simulink model "OMAP_ver_MIL10"  (R2018b)
settings: Solver=FixedStepDiscrete  StartTime=0.0  StopTime=10.0  FixedStep=0.01  RelTol=1e-3
undefined symbols (not defined in the file or in its folder): OMAP_Switch_EMS, OMAP_Switch_EPS, OMAP_Switch_ESC, OMAP_Switch_IC, OMAP_Switch_OTHER, TH_HMIClb_tiDgrdIconWarnHiDurT_C, TH_HMIClb_tiDgrdIconWarnLoDurT_C, TH_HMIClb_tiDgrdVocWarnDurT_C, TH_HMIClb_tiHndOffTxtWarnT_C, TH_HMIClb_tiHndOffVocWarnT_C, TH_HMIClb_tiSWALimFlgDetT_C, TH_HMIClb_tiTxtLimT_C
libraries: simulink x118
(part 5 of 9)

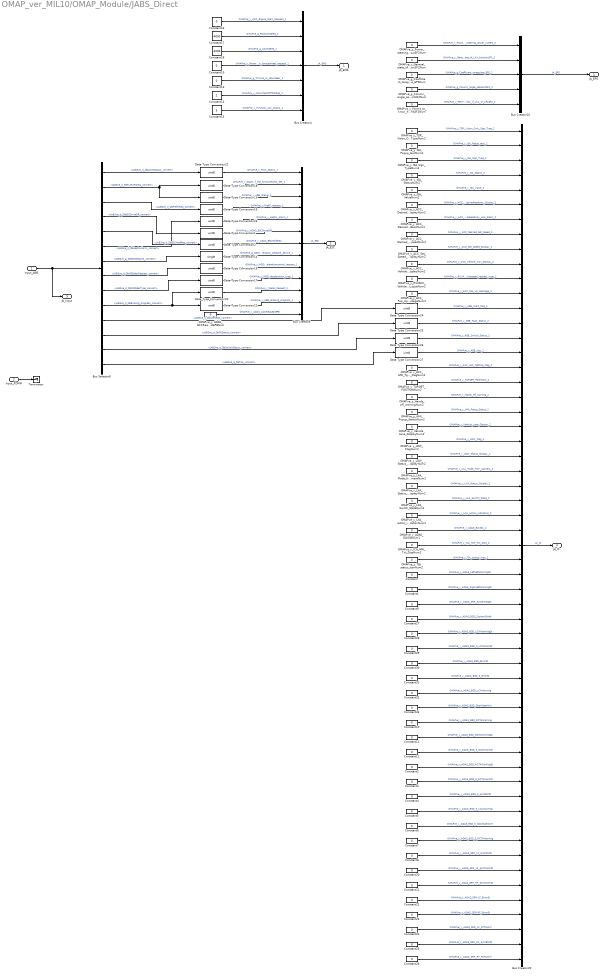
== system OMAP_ver_MIL10/OMAP_Module/JABS_Direct ==
  Input_JABS : Inport
  Input_FDMM : Inport  Port=2
  Bus Creator10 : BusCreator  Inputs=5
  Bus Creator20 : BusCreator  Inputs=57
  Bus Creator4 : BusCreator  Inputs=7
  Bus Creator9 : BusCreator  Inputs=13
  Bus Selector8 : BusSelector  OutputSignals=JABSve_d_DbJACWStatus_convert,JABSve_d_DbFunFARCSta_convert,JABSve_d_DbPrefillReq_convert,JABSve_d_DbESCDriveOff_convert,JABSve_d_DbESCHoldReq_convert,JABSve_d_DbHapticAlarm_convert,JABSve_g_DbDecSetpoint_convert,JABSve_d_DbMDDdecRequest_convert,JABSve_d_DbMDDdecType_convert,JABSve_d_DbBraking_progress_convert,JABSve_d_DbAlertReq_convert,JABSve_d_DbFltStatus_convert,JABSve_d_DbSwitchStatus_convert,JABSve_d_DbTips_convert
  Constant{,1..12,16,19..33} (29 alike) : Constant  Value=0  OutDataTypeStr=uint8
  Constant13 : Constant  Value=0  OutDataTypeStr=single
  Constant14 : Constant  Value=2  OutDataTypeStr=uint8
  Constant15 : Constant  Value=3  OutDataTypeStr=uint8
  Constant17 : Constant  Value=-4000  OutDataTypeStr=single
  Constant18 : Constant  Value=-4000  OutDataTypeStr=single
  Data Type Conversion{1..2,15..27} (15 alike) : DataTypeConversion  OutDataTypeStr=uint8
  Data Type Conversion14 : DataTypeConversion  OutDataTypeStr=single
  OMAPve_g_Coefficient_toregulate_EPSNum : Constant  Value=0  OutDataTypeStr=single
  OMAPve_g_Column_angle_setpoint3F2Num : Constant  Value=0  OutDataTypeStr=single
  OMAPve_y_ACC_DesiredHeadway_DisplayNum2 : Constant  Value=0  OutDataTypeStr=uint8
  OMAPve_y_ACC_DesiredHeadway_Icon_BasicNum2 : Constant  Value=0  OutDataTypeStr=uint8
  OMAPve_y_ACC_Desired_Set_SpeedNum2 : Constant  Value=0  OutDataTypeStr=uint8
  OMAPve_y_ACC_HMI_TgtDisp_FlagNum2 : Constant  Value=0  OutDataTypeStr=uint8
  OMAPve_y_ACC_Pop_Up_MessageNum2 : Constant  Value=0  OutDataTypeStr=uint8
  OMAPve_y_ACC_Set_Speed_DisplayNum2 : Constant  Value=0  OutDataTypeStr=uint8
  OMAPve_y_ACC_Vehicle_Icon_DisplayNum2 : Constant  Value=0  OutDataTypeStr=uint8
  OMAPve_y_ADAS_ACCRequestEPBNum : Constant  Value=0  OutDataTypeStr=uint8
  OMAPve_y_ADAS_ELKStsNum1 : Constant  Value=0  OutDataTypeStr=uint8
  OMAPve_y_General_state_of_LKA_function3F2Num : Constant  Value=0  OutDataTypeStr=uint8
  OMAPve_y_HMI_Popup_StatusNum2 : Constant  Value=0  OutDataTypeStr=uint8
  OMAPve_y_Hands_off_warningNum2 : Constant  Value=0  OutDataTypeStr=uint8
  OMAPve_y_ICA_HMI_Txt_DispNum2 : Constant  Value=0  OutDataTypeStr=uint8
  OMAPve_y_ISA_Popup_textNum2 : Constant  Value=0  OutDataTypeStr=uint8
  OMAPve_y_ISA_Sign_TypeNum2 : Constant  Value=0  OutDataTypeStr=uint8
  OMAPve_y_ISA_StatusNum2 : Constant  Value=0  OutDataTypeStr=uint8
  OMAPve_y_ISA_ValueNum2 : Constant  Value=0  OutDataTypeStr=uint8
  OMAPve_y_LDW_FlagNum2 : Constant  Value=0  OutDataTypeStr=uint8
  OMAPve_y_LDW_Status_DisplayNum2 : Constant  Value=0  OutDataTypeStr=uint8
  OMAPve_y_LKA_Mode_from_CameraNum2 : Constant  Value=0  OutDataTypeStr=uint8
  OMAPve_y_LKA_Status_DisplayNum2 : Constant  Value=0  OutDataTypeStr=uint8
  OMAPve_y_LKA_Switch_StateNum2 : Constant  Value=0  OutDataTypeStr=uint8
  OMAPve_y_LKA_action_indicationNum2 : Constant  Value=0  OutDataTypeStr=uint8
  OMAPve_y_Permit_to_know_if_LKA_or_LPA3F2Num : Constant  Value=0  OutDataTypeStr=uint8
  OMAPve_y_Power_steering_power_cut3F2Num : Constant  Value=0  OutDataTypeStr=uint8
  OMAPve_y_RVVACC_Vehiclespeed_request_typeNum2 : Constant  Value=0  OutDataTypeStr=uint8
  OMAPve_y_TARGET_POSITIONNum2 : Constant  Value=6  OutDataTypeStr=uint8
  OMAPve_y_TJA_status_iconNum2 : Constant  Value=0  OutDataTypeStr=uint8
  OMAPve_y_TSR_Vision_Only_Sign_TypeNum2 : Constant  Value=0  OutDataTypeStr=uint8
  OMAPve_y_Vehicle_Lane_DisplayNum2 : Constant  Value=0  OutDataTypeStr=uint8
  Terminator : Terminator
  JA_EMS : Outport
  JA_ESC : Outport  Port=2
  JA_EPS : Outport  Port=3
  JA_IC : Outport  Port=4
  JA_Input : Outport  Port=5
  wires:
  Bus Creator20/1 -> JA_IC/1  "JA_IC"
  OMAPve_y_ISA_StatusNum2/1 -> Bus Creator20/4  "OMAPve_y_ISA_Status_2"
  Bus Selector8/13 -> Data Type Conversion26/1  "<JABSve_d_DbSwitchStatus_convert>"
  Bus Selector8/14 -> Data Type Conversion27/1  "<JABSve_d_DbTips_convert>"
  Bus Selector8/9 -> Data Type Conversion17/1  "<JABSve_d_DbMDDdecType_convert>"
  Data Type Conversion27/1 -> Bus Creator20/16  "OMAPve_y_AEB_tips_2"
  OMAPve_y_ICA_HMI_Txt_DispNum2/1 -> Bus Creator20/29  "OMAPve_y_ICA_HMI_Txt_Disp_2"
  OMAPve_y_TARGET_POSITIONNum2/1 -> Bus Creator20/18  "OMAPve_y_TARGET_POSITION_2"
  OMAPve_y_ACC_Vehicle_Icon_DisplayNum2/1 -> Bus Creator20/10  "OMAPve_y_ACC_Vehicle_Icon_Display_2"
  Bus Selector8/6 -> Data Type Conversion23/1  "<JABSve_d_DbHapticAlarm_convert>"
  OMAPve_y_HMI_Popup_StatusNum2/1 -> Bus Creator20/20  "OMAPve_y_HMI_Popup_Status_2"
  OMAPve_y_LKA_Status_DisplayNum2/1 -> Bus Creator20/25  "OMAPve_y_LKA_Status_Display_2"
  OMAPve_y_ACC_DesiredHeadway_DisplayNum2/1 -> Bus Creator20/6  "OMAPve_y_ACC_DesiredHeadway_Display_2"
  Data Type Conversion25/1 -> Bus Creator20/14  "OMAPve_y_AEB_Fault_Status_2"
  Data Type Conversion24/1 -> Bus Creator20/13  "OMAPve_y_AEB_Alert_Req_2"
  OMAPve_y_ACC_HMI_TgtDisp_FlagNum2/1 -> Bus Creator20/17  "OMAPve_y_ACC_HMI_TgtDisp_Flag_2"
  Input_JABS/1 -> JA_Input/1, Bus Selector8/1
  OMAPve_y_ISA_Popup_textNum2/1 -> Bus Creator20/2  "OMAPve_y_ISA_Popup_text_2"
  OMAPve_y_LKA_Mode_from_CameraNum2/1 -> Bus Creator20/24  "OMAPve_y_LKA_Mode_from_Camera_2"
  OMAPve_y_ISA_Sign_TypeNum2/1 -> Bus Creator20/3  "OMAPve_y_ISA_Sign_Type_2"
  Bus Selector8/11 -> Data Type Conversion24/1  "<JABSve_d_DbAlertReq_convert>"
  OMAPve_y_Vehicle_Lane_DisplayNum2/1 -> Bus Creator20/21  "OMAPve_y_Vehicle_Lane_Display_2"
  OMAPve_y_LKA_action_indicationNum2/1 -> Bus Creator20/27  "OMAPve_y_LKA_action_indication_2"
  Bus Selector8/1 -> Data Type Conversion22/1  "<JABSve_d_DbJACWStatus_convert>"
  Data Type Conversion15/1 -> Bus Creator9/9  "OMAPve_y_MDD_Decelerationcontrol_request_1"
  OMAPve_y_ACC_Desired_Set_SpeedNum2/1 -> Bus Creator20/8  "OMAPve_y_ACC_Desired_Set_Speed_2"
  OMAPve_y_TSR_Vision_Only_Sign_TypeNum2/1 -> Bus Creator20/1  "OMAPve_y_TSR_Vision_Only_Sign_Type_2"
  Constant15/1 -> Bus Creator4/7  "OMAPve_y_Function_Acc_status_1"
  Bus Creator4/1 -> JA_EMS/1  "JA_EMS"
  Constant13/1 -> Bus Creator4/5  "OMAPve_g_TminUp_or_downGear_1"
  Bus Selector8/12 -> Data Type Conversion25/1  "<JABSve_d_DbFltStatus_convert>"
  OMAPve_y_LDW_Status_DisplayNum2/1 -> Bus Creator20/23  "OMAPve_y_LDW_Status_Display_2"
  Data Type Conversion26/1 -> Bus Creator20/15  "OMAPve_y_AEB_Switch_Status_2"
  Data Type Conversion22/1 -> Bus Creator9/1  "OMAPve_y_FCW_Status_1"
  Data Type Conversion17/1 -> Bus Creator9/10  "OMAPve_y_MDD_deceleration_type_1"
  Data Type Conversion14/1 -> Bus Creator9/8  "OMAPve_g_Deceleration_setpoint_device_1"
  Bus Selector8/3 -> Data Type Conversion16/1  "<JABSve_d_DbPrefillReq_convert>"
  Constant14/1 -> Bus Creator4/6  "OMAPve_y_stAcvTqWhlPTPotReq_1"
  Bus Selector8/8 -> Data Type Conversion15/1  "<JABSve_d_DbMDDdecRequest_convert>"
  Bus Creator9/1 -> JA_ESC/1  "JA_ESC"
  Constant16/1 -> Bus Creator4/1  "OMAPve_y_ACC_Engine_Start_Request_1"
  OMAPve_y_LKA_Switch_StateNum2/1 -> Bus Creator20/26  "OMAPve_y_LKA_Switch_State_2"
  OMAPve_y_ACC_DesiredHeadway_Icon_BasicNum2/1 -> Bus Creator20/7  "OMAPve_y_ACC_DesiredHeadway_Icon_Basic_2"
  OMAPve_y_LDW_FlagNum2/1 -> Bus Creator20/22  "OMAPve_y_LDW_Flag_2"
  Data Type Conversion16/1 -> Bus Creator9/4  "OMAPve_y_Prefill_request_1"
  Data Type Conversion18/1 -> Bus Creator9/2  "OMAPve_y_State_of_the_functionFARC_det_1"
  Constant19/1 -> Bus Creator4/4  "OMAPve_y_Powertrain_torquewheel_request_1"
  OMAPve_y_ISA_ValueNum2/1 -> Bus Creator20/5  "OMAPve_y_ISA_Value_2"
  Data Type Conversion23/1 -> Bus Creator9/5  "OMAPve_y_Haptic_Alarm_1"
  Data Type Conversion19/1 -> Bus Creator9/3  "OMAPve_y_AEB_Status_1"
  OMAPve_y_RVVACC_Vehiclespeed_request_typeNum2/1 -> Bus Creator20/11  "OMAPve_y_RVVACC_Vehiclespeed_request_type_2"
  Bus Selector8/7 -> Data Type Conversion14/1  "<JABSve_g_DbDecSetpoint_convert>"
  Constant18/1 -> Bus Creator4/3  "OMAPve_g_ACCTqReq_1"
  OMAPve_y_Hands_off_warningNum2/1 -> Bus Creator20/19  "OMAPve_y_Hands_off_warning_2"
  OMAPve_y_TJA_status_iconNum2/1 -> Bus Creator20/30  "OMAPve_y_TJA_status_icon_2"
  Constant17/1 -> Bus Creator4/2  "OMAPve_g_PotACCTqReq_1"
  OMAPve_y_ACC_Pop_Up_MessageNum2/1 -> Bus Creator20/12  "OMAPve_y_ACC_Pop_Up_Message_2"
  Bus Selector8/2 -> Data Type Conversion18/1, Data Type Conversion19/1  "<JABSve_d_DbFunFARCSta_convert>"
  Data Type Conversion20/1 -> Bus Creator9/11  "OMAPve_y_Decel_Request_1"
  OMAPve_y_ACC_Set_Speed_DisplayNum2/1 -> Bus Creator20/9  "OMAPve_y_ACC_Set_Speed_Display_2"
  Data Type Conversion21/1 -> Bus Creator9/12  "OMAPve_y_AEB_Braking_progress_1"
  OMAPve_y_Power_steering_power_cut3F2Num/1 -> Bus Creator10/1  "OMAPve_y_Power_steering_power_cut3F2_2"
  Bus Creator10/1 -> JA_EPS/1  "JA_EPS"
  OMAPve_y_Permit_to_know_if_LKA_or_LPA3F2Num/1 -> Bus Creator10/5  "OMAPve_y_Permit_to_know_if_LKA_or_LPA3F2_2"
  OMAPve_g_Coefficient_toregulate_EPSNum/1 -> Bus Creator10/3  "OMAPve_g_Coefficient_toregulate_EPS_2"
  OMAPve_y_General_state_of_LKA_function3F2Num/1 -> Bus Creator10/2  "OMAPve_y_General_state_of_LKA_function3F2_2"
  OMAPve_g_Column_angle_setpoint3F2Num/1 -> Bus Creator10/4  "OMAPve_g_Column_angle_setpoint3F2_2"
  Bus Selector8/10 -> Data Type Conversion20/1, Data Type Conversion21/1  "<JABSve_d_DbBraking_progress_convert>"
  Input_FDMM/1 -> Terminator/1
  OMAPve_y_ADAS_ELKStsNum1/1 -> Bus Creator20/28  "OMAPve_y_ADAS_ELKSts_2"
  Data Type Conversion2/1 -> Bus Creator9/7  "OMAPve_y_ADAS_ESCHoldReq"
  Data Type Conversion1/1 -> Bus Creator9/6  "OMAPve_y_ADAS_ESCDriveOff"
  OMAPve_y_ADAS_ACCRequestEPBNum/1 -> Bus Creator9/13  "OMAPve_y_ADAS_ACCRequestEPB"
  Constant6/1 -> Bus Creator20/48  "OMAPve_y_ADAS_BSD_S_DoorOpenWrn"
  Constant5/1 -> Bus Creator20/47  "OMAPve_y_ADAS_BSD_S_LCAWarning"
  Constant1/1 -> Bus Creator20/32  "OMAPve_y_ADAS_RighrLEDWarningSt"
  Constant8/1 -> Bus Creator20/50  "OMAPve_y_ADAS_SRR_LF_SystStInfo"
  Constant10/1 -> Bus Creator20/41  "OMAPve_y_ADAS_BSD_RCTAWarning"
  Constant33/1 -> Bus Creator20/40  "OMAPve_y_ADAS_BSD_DoorOpenWrn"
  Constant22/1 -> Bus Creator20/53  "OMAPve_y_ADAS_SRR-LF_ErrorSt"
  Constant7/1 -> Bus Creator20/49  "OMAPve_y_ADAS_BSD_S_RCTAWarning"
  Constant20/1 -> Bus Creator20/51  "OMAPve_y_ADAS_SRR_LF_SystWorkSt"
  Constant21/1 -> Bus Creator20/52  "OMAPve_y_ADAS_SRR_RF_SystWorkSt"
  Constant4/1 -> Bus Creator20/46  "OMAPve_y_ADAS_BSD_S_SystStInfo"
  Constant3/1 -> Bus Creator20/45  "OMAPve_y_ADAS_BSD_S_RCTAWorkSt"
  Constant2/1 -> Bus Creator20/44  "OMAPve_y_ADAS_BSD_RCTAWorkingSt"
  Constant23/1 -> Bus Creator20/54  "OMAPve_y_ADAS_SRR-RF_ErrorSt"
  Constant26/1 -> Bus Creator20/57  "OMAPve_y_ADAS_SRR_RF_FCTAWrn"
  Constant/1 -> Bus Creator20/31  "OMAPve_y_ADAS_LeftLEDWarningSt"
  Constant25/1 -> Bus Creator20/56  "OMAPve_y_ADAS_SRR_RF_SystStInfo"
  Constant24/1 -> Bus Creator20/55  "OMAPve_y_ADAS_SRR_LF_FCTAWrn"
  Constant28/1 -> Bus Creator20/35  "OMAPve_y_ADAS_BSD_LCWWorkingSt"
  Constant32/1 -> Bus Creator20/39  "OMAPve_y_ADAS_BSD_LCAWarning"
  Constant12/1 -> Bus Creator20/43  "OMAPve_y_ADAS_BSD_S_DOWWorkSt"
  Constant29/1 -> Bus Creator20/36  "OMAPve_y_ADAS_BSD_S_LCWWorkSt"
  Constant31/1 -> Bus Creator20/38  "OMAPve_y_ADAS_BSD_S_ErrorSt"
  Constant9/1 -> Bus Creator20/33  "OMAPve_y_ADAS_SRR_SystemState"
  Constant30/1 -> Bus Creator20/37  "OMAPve_y_ADAS_BSD_ErrorSt"
  Constant27/1 -> Bus Creator20/34  "OMAPve_y_ADAS_BSD_SystemStInfo"
  Constant11/1 -> Bus Creator20/42  "OMAPve_y_ADAS_BSD_DOWWorkingSt"
  Bus Selector8/4 -> Data Type Conversion1/1  "<JABSve_d_DbESCDriveOff_convert>"
  Bus Selector8/5 -> Data Type Conversion2/1  "<JABSve_d_DbESCHoldReq_convert>"

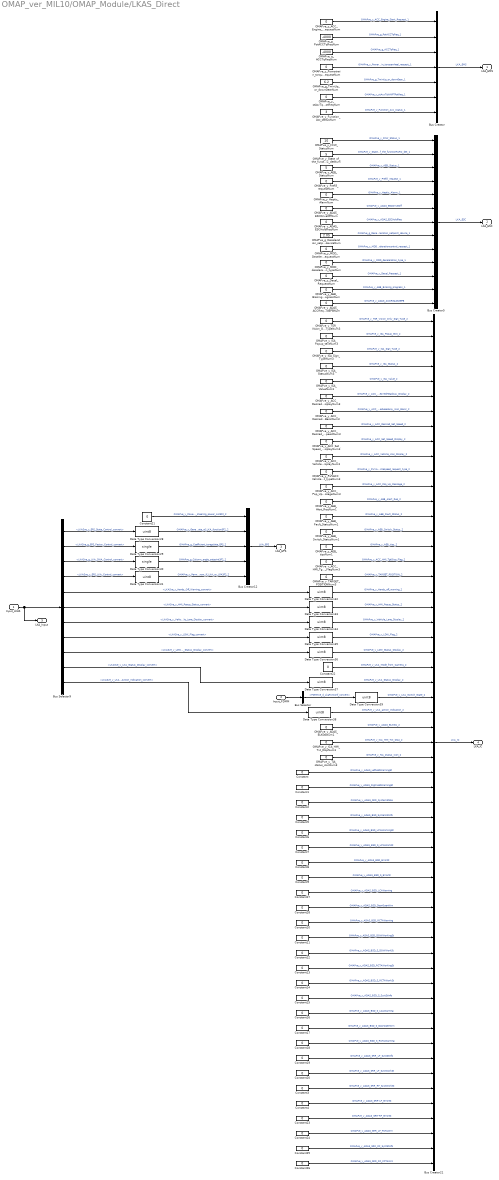
== system OMAP_ver_MIL10/OMAP_Module/LKAS_Direct ==
  Input_LKAS : Inport
  Input_FDMM : Inport  Port=2
  Bus Creator : BusCreator  Inputs=7
  Bus Creator12 : BusCreator  Inputs=5
  Bus Creator21 : BusCreator  Inputs=57
  Bus Creator5 : BusCreator  Inputs=13
  Bus Selector : BusSelector  OutputSignals=FDMMve_d_LkaFcnConf_convert
  Bus Selector9 : BusSelector  OutputSignals=LKASve_y_EPS_State_Control_convert,LKASve_g_EPS_Factor_Control_convert,LKASve_g_LKA_SWA_Control_convert,LKASve_y_EPS_LKA_Control_convert,LKASve_y_Hands_Off_Warning_convert,LKASve_y_HMI_Popup_Status_convert,LKASve_y_Vehicle_Lane_Display_convert,LKASve_y_LDW_Flag_convert,LKASve_y_LDW_Status_Display_convert,LKASve_y_LKA_Status_Display_convert,LKASve_y_LKA_Action_Indication_convert
  Constant{,1..28} (29 alike) : Constant  Value=0  OutDataTypeStr=uint8
  Data Type Conversion{28,31..39} (10 alike) : DataTypeConversion  OutDataTypeStr=uint8
  Data Type Conversion29 : DataTypeConversion  OutDataTypeStr=single
  Data Type Conversion30 : DataTypeConversion  OutDataTypeStr=single
  OMAPve_g_ACCTqReqNum : Constant  Value=-4000  OutDataTypeStr=single
  OMAPve_g_Deceleration_setpoint_deviceNum : Constant  Value=2.05  OutDataTypeStr=single
  OMAPve_g_PotACCTqReqNum : Constant  Value=-4000  OutDataTypeStr=single
  OMAPve_g_TminUp_or_downGearNum : Constant  Value=6.2  OutDataTypeStr=single
  OMAPve_y_ACC_DesiredHeadway_DisplayNum3 : Constant  Value=0  OutDataTypeStr=uint8
  OMAPve_y_ACC_DesiredHeadway_Icon_BasicNum3 : Constant  Value=0  OutDataTypeStr=uint8
  OMAPve_y_ACC_Desired_Set_SpeedNum3 : Constant  Value=0  OutDataTypeStr=uint8
  OMAPve_y_ACC_Engine_Start_RequestNum : Constant  Value=0  OutDataTypeStr=uint8
  OMAPve_y_ACC_HMI_TgtDisp_FlagNum3 : Constant  Value=0  OutDataTypeStr=uint8
  OMAPve_y_ACC_Pop_Up_MessageNum3 : Constant  Value=0  OutDataTypeStr=uint8
  OMAPve_y_ACC_Set_Speed_DisplayNum3 : Constant  Value=0  OutDataTypeStr=uint8
  OMAPve_y_ACC_Vehicle_Icon_DisplayNum3 : Constant  Value=0  OutDataTypeStr=uint8
  OMAPve_y_ADAS_ACCRequestEPBNum : Constant  Value=0  OutDataTypeStr=uint8
  OMAPve_y_ADAS_ELKStsNum1 : Constant  Value=0  OutDataTypeStr=uint8
  OMAPve_y_ADAS_ESCDriveOffNum : Constant  Value=0  OutDataTypeStr=uint8
  OMAPve_y_ADAS_ESCHoldReqNum : Constant  Value=0  OutDataTypeStr=uint8
  OMAPve_y_AEB_Alert_ReqNum1 : Constant  Value=0  OutDataTypeStr=uint8
  OMAPve_y_AEB_Braking_progressNum : Constant  Value=0  OutDataTypeStr=uint8
  OMAPve_y_AEB_Fault_StatusNum1 : Constant  Value=0  OutDataTypeStr=uint8
  OMAPve_y_AEB_StatusNum : Constant  Value=5  OutDataTypeStr=uint8
  OMAPve_y_AEB_Switch_StatusNum1 : Constant  Value=0  OutDataTypeStr=uint8
  OMAPve_y_AEB_tipsNum1 : Constant  Value=0  OutDataTypeStr=uint8
  OMAPve_y_Decel_RequestNum : Constant  Value=0  OutDataTypeStr=uint8
  OMAPve_y_FCW_StatusNum : Constant  Value=10  OutDataTypeStr=uint8
  OMAPve_y_Function_Acc_statusNum : Constant  Value=3  OutDataTypeStr=uint8
  OMAPve_y_Haptic_AlarmNum : Constant  Value=0  OutDataTypeStr=uint8
  OMAPve_y_ICA_HMI_Txt_DispNum3 : Constant  Value=0  OutDataTypeStr=uint8
  OMAPve_y_ISA_Popup_textNum3 : Constant  Value=0  OutDataTypeStr=uint8
  OMAPve_y_ISA_Sign_TypeNum3 : Constant  Value=0  OutDataTypeStr=uint8
  OMAPve_y_ISA_StatusNum3 : Constant  Value=0  OutDataTypeStr=uint8
  OMAPve_y_ISA_ValueNum3 : Constant  Value=0  OutDataTypeStr=uint8
  OMAPve_y_MDD_Decelerationcontrol_requestNum : Constant  Value=0  OutDataTypeStr=uint8
  OMAPve_y_MDD_deceleration_typeNum : Constant  Value=0  OutDataTypeStr=uint8
  OMAPve_y_Powertrain_torquewheel_requestNum : Constant  Value=0  OutDataTypeStr=uint8
  OMAPve_y_Prefill_requestNum : Constant  Value=0  OutDataTypeStr=uint8
  OMAPve_y_RVVACC_Vehiclespeed_request_typeNum3 : Constant  Value=0  OutDataTypeStr=uint8
  OMAPve_y_State_of_the_functionFARC_detNum : Constant  Value=5  OutDataTypeStr=uint8
  OMAPve_y_TARGET_POSITIONNum3 : Constant  Value=6  OutDataTypeStr=uint8
  OMAPve_y_TJA_status_iconNum3 : Constant  Value=0  OutDataTypeStr=uint8
  OMAPve_y_TSR_Vision_Only_Sign_TypeNum3 : Constant  Value=0  OutDataTypeStr=uint8
  OMAPve_y_stAcvTqWhlPTPotReqNum : Constant  Value=0  OutDataTypeStr=uint8
  LKA_EMS : Outport
  LKA_ESC : Outport  Port=2
  LKA_EPS : Outport  Port=3
  LKA_IC : Outport  Port=4
  LKA_Input : Outport  Port=5
  wires:
  Bus Selector/1 -> Data Type Conversion39/1  "<FDMMve_d_LkaFcnConf_convert>"
  Bus Selector9/11 -> Data Type Conversion38/1  "<LKASve_y_LKA_Action_Indication_convert>"
  Bus Selector9/4 -> Data Type Conversion31/1  "<LKASve_y_EPS_LKA_Control_convert>"
  OMAPve_y_TSR_Vision_Only_Sign_TypeNum3/1 -> Bus Creator21/1  "OMAPve_y_TSR_Vision_Only_Sign_Type_2"
  Bus Selector9/5 -> Data Type Conversion32/1  "<LKASve_y_Hands_Off_Warning_convert>"
  Data Type Conversion39/1 -> Bus Creator21/26  "OMAPve_y_LKA_Switch_State_2"
  Data Type Conversion34/1 -> Bus Creator21/21  "OMAPve_y_Vehicle_Lane_Display_2"
  Bus Selector9/10 -> Data Type Conversion37/1  "<LKASve_y_LKA_Status_Display_convert>"
  Bus Creator12/1 -> LKA_EPS/1  "LKA_EPS"
  Bus Selector9/6 -> Data Type Conversion33/1  "<LKASve_y_HMI_Popup_Status_convert>"
  Data Type Conversion32/1 -> Bus Creator21/19  "OMAPve_y_Hands_off_warning_2"
  Input_FDMM/1 -> Bus Selector/1
  Constant22/1 -> Bus Creator21/24  "OMAPve_y_LKA_Mode_from_Camera_2"
  OMAPve_y_ISA_Popup_textNum3/1 -> Bus Creator21/2  "OMAPve_y_ISA_Popup_text_2"
  Constant21/1 -> Bus Creator12/1  "OMAPve_y_Power_steering_power_cut3F2_2"
  OMAPve_y_TJA_status_iconNum3/1 -> Bus Creator21/30  "OMAPve_y_TJA_status_icon_2"
  Data Type Conversion29/1 -> Bus Creator12/3  "OMAPve_g_Coefficient_toregulate_EPS_2"
  Input_LKAS/1 -> LKA_Input/1, Bus Selector9/1
  OMAPve_y_ACC_DesiredHeadway_DisplayNum3/1 -> Bus Creator21/6  "OMAPve_y_ACC_DesiredHeadway_Display_2"
  OMAPve_y_ACC_Pop_Up_MessageNum3/1 -> Bus Creator21/12  "OMAPve_y_ACC_Pop_Up_Message_2"
  OMAPve_y_ACC_Vehicle_Icon_DisplayNum3/1 -> Bus Creator21/10  "OMAPve_y_ACC_Vehicle_Icon_Display_2"
  Bus Selector9/8 -> Data Type Conversion35/1  "<LKASve_y_LDW_Flag_convert>"
  OMAPve_y_ICA_HMI_Txt_DispNum3/1 -> Bus Creator21/29  "OMAPve_y_ICA_HMI_Txt_Disp_2"
  OMAPve_y_TARGET_POSITIONNum3/1 -> Bus Creator21/18  "OMAPve_y_TARGET_POSITION_2"
  Data Type Conversion37/1 -> Bus Creator21/25  "OMAPve_y_LKA_Status_Display_2"
  OMAPve_y_RVVACC_Vehiclespeed_request_typeNum3/1 -> Bus Creator21/11  "OMAPve_y_RVVACC_Vehiclespeed_request_type_2"
  Data Type Conversion36/1 -> Bus Creator21/23  "OMAPve_y_LDW_Status_Display_2"
  Data Type Conversion38/1 -> Bus Creator21/27  "OMAPve_y_LKA_action_indication_2"
  OMAPve_y_AEB_Switch_StatusNum1/1 -> Bus Creator21/15  "OMAPve_y_AEB_Switch_Status_2"
  Bus Selector9/2 -> Data Type Conversion29/1  "<LKASve_g_EPS_Factor_Control_convert>"
  Data Type Conversion33/1 -> Bus Creator21/20  "OMAPve_y_HMI_Popup_Status_2"
  OMAPve_y_ISA_Sign_TypeNum3/1 -> Bus Creator21/3  "OMAPve_y_ISA_Sign_Type_2"
  OMAPve_y_ISA_ValueNum3/1 -> Bus Creator21/5  "OMAPve_y_ISA_Value_2"
  OMAPve_y_AEB_Fault_StatusNum1/1 -> Bus Creator21/14  "OMAPve_y_AEB_Fault_Status_2"
  OMAPve_y_ACC_Set_Speed_DisplayNum3/1 -> Bus Creator21/9  "OMAPve_y_ACC_Set_Speed_Display_2"
  Bus Selector9/1 -> Data Type Conversion28/1  "<LKASve_y_EPS_State_Control_convert>"
  Bus Creator21/1 -> LKA_IC/1  "LKA_IC"
  OMAPve_y_ACC_HMI_TgtDisp_FlagNum3/1 -> Bus Creator21/17  "OMAPve_y_ACC_HMI_TgtDisp_Flag_2"
  OMAPve_y_ISA_StatusNum3/1 -> Bus Creator21/4  "OMAPve_y_ISA_Status_2"
  Data Type Conversion28/1 -> Bus Creator12/2  "OMAPve_y_General_state_of_LKA_function3F2_2"
  Bus Selector9/7 -> Data Type Conversion34/1  "<LKASve_y_Vehicle_Lane_Display_convert>"
  Data Type Conversion31/1 -> Bus Creator12/5  "OMAPve_y_Permit_to_know_if_LKA_or_LPA3F2_2"
  OMAPve_y_ACC_DesiredHeadway_Icon_BasicNum3/1 -> Bus Creator21/7  "OMAPve_y_ACC_DesiredHeadway_Icon_Basic_2"
  Data Type Conversion35/1 -> Bus Creator21/22  "OMAPve_y_LDW_Flag_2"
  OMAPve_y_ACC_Desired_Set_SpeedNum3/1 -> Bus Creator21/8  "OMAPve_y_ACC_Desired_Set_Speed_2"
  Data Type Conversion30/1 -> Bus Creator12/4  "OMAPve_g_Column_angle_setpoint3F2_2"
  Bus Selector9/3 -> Data Type Conversion30/1  "<LKASve_g_LKA_SWA_Control_convert>"
  Bus Selector9/9 -> Data Type Conversion36/1  "<LKASve_y_LDW_Status_Display_convert>"
  OMAPve_y_AEB_tipsNum1/1 -> Bus Creator21/16  "OMAPve_y_AEB_tips_2"
  OMAPve_y_AEB_Alert_ReqNum1/1 -> Bus Creator21/13  "OMAPve_y_AEB_Alert_Req_2"
  OMAPve_g_TminUp_or_downGearNum/1 -> Bus Creator/5  "OMAPve_g_TminUp_or_downGear_1"
  Bus Creator/1 -> LKA_EMS/1  "LKA_EMS"
  OMAPve_g_PotACCTqReqNum/1 -> Bus Creator/2  "OMAPve_g_PotACCTqReq_1"
  OMAPve_y_Powertrain_torquewheel_requestNum/1 -> Bus Creator/4  "OMAPve_y_Powertrain_torquewheel_request_1"
  OMAPve_g_ACCTqReqNum/1 -> Bus Creator/3  "OMAPve_g_ACCTqReq_1"
  OMAPve_y_ACC_Engine_Start_RequestNum/1 -> Bus Creator/1  "OMAPve_y_ACC_Engine_Start_Request_1"
  OMAPve_y_Function_Acc_statusNum/1 -> Bus Creator/7  "OMAPve_y_Function_Acc_status_1"
  OMAPve_y_stAcvTqWhlPTPotReqNum/1 -> Bus Creator/6  "OMAPve_y_stAcvTqWhlPTPotReq_1"
  OMAPve_y_MDD_deceleration_typeNum/1 -> Bus Creator5/10  "OMAPve_y_MDD_deceleration_type_1"
  OMAPve_y_MDD_Decelerationcontrol_requestNum/1 -> Bus Creator5/9  "OMAPve_y_MDD_Decelerationcontrol_request_1"
  OMAPve_y_Decel_RequestNum/1 -> Bus Creator5/11  "OMAPve_y_Decel_Request_1"
  OMAPve_y_Prefill_requestNum/1 -> Bus Creator5/4  "OMAPve_y_Prefill_request_1"
  OMAPve_g_Deceleration_setpoint_deviceNum/1 -> Bus Creator5/8  "OMAPve_g_Deceleration_setpoint_device_1"
  OMAPve_y_AEB_StatusNum/1 -> Bus Creator5/3  "OMAPve_y_AEB_Status_1"
  OMAPve_y_AEB_Braking_progressNum/1 -> Bus Creator5/12  "OMAPve_y_AEB_Braking_progress_1"
  OMAPve_y_FCW_StatusNum/1 -> Bus Creator5/1  "OMAPve_y_FCW_Status_1"
  OMAPve_y_State_of_the_functionFARC_detNum/1 -> Bus Creator5/2  "OMAPve_y_State_of_the_functionFARC_det_1"
  OMAPve_y_Haptic_AlarmNum/1 -> Bus Creator5/5  "OMAPve_y_Haptic_Alarm_1"
  Bus Creator5/1 -> LKA_ESC/1  "LKA_ESC"
  OMAPve_y_ADAS_ELKStsNum1/1 -> Bus Creator21/28  "OMAPve_y_ADAS_ELKSts_2"
  OMAPve_y_ADAS_ESCHoldReqNum/1 -> Bus Creator5/7  "OMAPve_y_ADAS_ESCHoldReq"
  OMAPve_y_ADAS_ESCDriveOffNum/1 -> Bus Creator5/6  "OMAPve_y_ADAS_ESCDriveOff"
  OMAPve_y_ADAS_ACCRequestEPBNum/1 -> Bus Creator5/13  "OMAPve_y_ADAS_ACCRequestEPB"
  Constant17/1 -> Bus Creator21/48  "OMAPve_y_ADAS_BSD_S_DoorOpenWrn"
  Constant16/1 -> Bus Creator21/47  "OMAPve_y_ADAS_BSD_S_LCAWarning"
  Constant1/1 -> Bus Creator21/32  "OMAPve_y_ADAS_RighrLEDWarningSt"
  Constant19/1 -> Bus Creator21/50  "OMAPve_y_ADAS_SRR_LF_SystStInfo"
  Constant10/1 -> Bus Creator21/41  "OMAPve_y_ADAS_BSD_RCTAWarning"
  Constant28/1 -> Bus Creator21/40  "OMAPve_y_ADAS_BSD_DoorOpenWrn"
  Constant4/1 -> Bus Creator21/53  "OMAPve_y_ADAS_SRR-LF_ErrorSt"
  Constant18/1 -> Bus Creator21/49  "OMAPve_y_ADAS_BSD_S_RCTAWarning"
  Constant20/1 -> Bus Creator21/51  "OMAPve_y_ADAS_SRR_LF_SystWorkSt"
  Constant3/1 -> Bus Creator21/52  "OMAPve_y_ADAS_SRR_RF_SystWorkSt"
  Constant15/1 -> Bus Creator21/46  "OMAPve_y_ADAS_BSD_S_SystStInfo"
  Constant14/1 -> Bus Creator21/45  "OMAPve_y_ADAS_BSD_S_RCTAWorkSt"
  Constant13/1 -> Bus Creator21/44  "OMAPve_y_ADAS_BSD_RCTAWorkingSt"
  Constant23/1 -> Bus Creator21/54  "OMAPve_y_ADAS_SRR-RF_ErrorSt"
  Constant26/1 -> Bus Creator21/57  "OMAPve_y_ADAS_SRR_RF_FCTAWrn"
  Constant/1 -> Bus Creator21/31  "OMAPve_y_ADAS_LeftLEDWarningSt"
  Constant25/1 -> Bus Creator21/56  "OMAPve_y_ADAS_SRR_RF_SystStInfo"
  Constant24/1 -> Bus Creator21/55  "OMAPve_y_ADAS_SRR_LF_FCTAWrn"
  Constant6/1 -> Bus Creator21/35  "OMAPve_y_ADAS_BSD_LCWWorkingSt"
  Constant27/1 -> Bus Creator21/39  "OMAPve_y_ADAS_BSD_LCAWarning"
  Constant12/1 -> Bus Creator21/43  "OMAPve_y_ADAS_BSD_S_DOWWorkSt"
  Constant7/1 -> Bus Creator21/36  "OMAPve_y_ADAS_BSD_S_LCWWorkSt"
  Constant9/1 -> Bus Creator21/38  "OMAPve_y_ADAS_BSD_S_ErrorSt"
  Constant2/1 -> Bus Creator21/33  "OMAPve_y_ADAS_SRR_SystemState"
  Constant8/1 -> Bus Creator21/37  "OMAPve_y_ADAS_BSD_ErrorSt"
  Constant5/1 -> Bus Creator21/34  "OMAPve_y_ADAS_BSD_SystemStInfo"
  Constant11/1 -> Bus Creator21/42  "OMAPve_y_ADAS_BSD_DOWWorkingSt"

== system OMAP_ver_MIL10/OMAP_Module/OTHER_Default_Arbitration ==
  Bus Creator27 : BusCreator  Inputs=5
  Data Type Conversion72 : DataTypeConversion  OutDataTypeStr=uint8
  Delay : Delay
  NOT : Logic  Operator=NOT  IconShape=distinctive  AllPortsSameDT=off  OutDataTypeStr=boolean
  OMAPve_y_ABS_ESP_power_cut_request2Num1 : Constant  Value=0  OutDataTypeStr=uint8
  OMAPve_y_ASR_connection_dis_demand2Num1 : Constant  Value=0  OutDataTypeStr=uint8
  OMAPve_y_ECU_operating_phaseNum1 : Constant  Value=9  OutDataTypeStr=uint8
  OMAPve_y_Radar_StateNum1 : Constant  Value=2  OutDataTypeStr=uint8
  Arbitration : Outport
  wires:
  Bus Creator27/1 -> Arbitration/1  "Arbitration"
  Data Type Conversion72/1 -> Bus Creator27/3  "OMAPve_y_TYPE_RAPPORT_2"
  Delay/1 -> NOT/1
  OMAPve_y_ASR_connection_dis_demand2Num1/1 -> Bus Creator27/2  "OMAPve_y_ASR_connection_dis_demand2_2"
  OMAPve_y_ABS_ESP_power_cut_request2Num1/1 -> Bus Creator27/1  "OMAPve_y_ABS_ESP_power_cut_request2_2"
  OMAPve_y_ECU_operating_phaseNum1/1 -> Bus Creator27/4  "OMAPve_y_ECU_operating_phase_2"
  OMAPve_y_Radar_StateNum1/1 -> Bus Creator27/5  "OMAPve_y_Radar_State_2"
  NOT/1 -> Delay/1, Data Type Conversion72/1

== system OMAP_ver_MIL10/OMAP_Module/ACCS_Direct/ACCS_Define ==
  In1 : Inport
  In2 : Inport  Port=2
  In3 : Inport  Port=3
  ACC_State_Synthesis(ACC_SS) : Subsystem
  Bus Creator : BusCreator  Inputs=11
  Bus Selector1 : BusSelector  OutputSignals=ACCSve_d_CIPV_ID_convert,ACCSve_d_ACC_State_convert,ACCSve_d_ACCActive_Signal_convert,ACCSve_d_ACC_ICA_Flag_convert,ACCSve_d_HeadWaySet_convert,ACCSve_d_VelocitySet_convert,ACCSve_d_ACC_go_request_convert,ACCSve_g_ACC_DecReq_convert
  Bus Selector2 : BusSelector  OutputSignals=IMAPva_d_obj_id_convert,IMAPva_g_obj_pos_x_convert
  CIPV_Data : MATLAB Function  TreatAsAtomicUnit=on
  Human_Machine_Interface(ACC_HMI) : Subsystem
  Terminator1 : Terminator
  Out1 : Outport
  Out2 : Outport  Port=2
  wires:
  ACC_State_Synthesis(ACC_SS)/1(ACC_Control_Signal) -> Out1/1
  In2/1 -> Terminator1/1
  In1/1 -> Bus Selector1/1, ACC_State_Synthesis(ACC_SS)/1(Input_ACCS)
  Human_Machine_Interface(ACC_HMI)/1(ACC_DesiredHeadway_Display) -> Bus Creator/1  "OMAPve_y_ACC_DesiredHeadway_Display_2"
  Human_Machine_Interface(ACC_HMI)/2(ACC_DesiredHeadway_Icon_Basic) -> Bus Creator/2  "OMAPve_y_ACC_DesiredHeadway_Icon_Basic_2"
  Human_Machine_Interface(ACC_HMI)/3(ACC_Desired_Set_Speed) -> Bus Creator/3  "OMAPve_y_ACC_Desired_Set_Speed_2"
  Human_Machine_Interface(ACC_HMI)/4(ACC_Set_Speed_Display) -> Bus Creator/4  "OMAPve_y_ACC_Set_Speed_Display_2"
  Human_Machine_Interface(ACC_HMI)/5(ACC_Vehicle_Icon_Display) -> Bus Creator/5  "OMAPve_y_ACC_Vehicle_Icon_Display_2"
  Human_Machine_Interface(ACC_HMI)/6(RVVACC_Vehiclespeed_request_type) -> Bus Creator/6  "OMAPve_y_RVVACC_Vehiclespeed_request_type_2"
  Human_Machine_Interface(ACC_HMI)/7(ACC_Pop_Up_Message) -> Bus Creator/7  "OMAPve_y_ACC_Pop_Up_Message_2"
  Human_Machine_Interface(ACC_HMI)/8(ACC_HMI_TgDisp_Flag) -> Bus Creator/8  "OMAPve_y_ACC_HMI_TgtDisp_Flag_2"
  Human_Machine_Interface(ACC_HMI)/9(TARGET_POSITION) -> Bus Creator/9  "OMAPve_y_TARGET_POSITION_2"
  Human_Machine_Interface(ACC_HMI)/10(ACC_Pop_Up_Message_TJA) -> Bus Creator/10  "ACC_Pop_Up_Message_TJA"
  Bus Creator/1 -> Out2/1
  Bus Selector1/7 -> Human_Machine_Interface(ACC_HMI)/8(ACC_go_request)  "<ACCSve_d_ACC_go_request_convert>"
  Bus Selector1/4 -> Human_Machine_Interface(ACC_HMI)/5(ACC_ICA_Flag)  "<ACCSve_d_ACC_ICA_Flag_convert>"
  Bus Selector1/1 -> Human_Machine_Interface(ACC_HMI)/2(CIPV_ID), CIPV_Data/3(ACCSve_d_CIPV_ID)  "<ACCSve_d_CIPV_ID_convert>"
  Bus Selector1/5 -> Human_Machine_Interface(ACC_HMI)/6(HeadWaySet)  "<ACCSve_d_HeadWaySet_convert>"
  CIPV_Data/1(CIPV_ID_Longitudinal_Distance) -> Human_Machine_Interface(ACC_HMI)/1(CIPV_ID_Longitudinal_Distance)
  Bus Selector1/3 -> Human_Machine_Interface(ACC_HMI)/4(ACCActive_Signal)  "<ACCSve_d_ACCActive_Signal_convert>"
  Bus Selector1/2 -> Bus Creator/11, Human_Machine_Interface(ACC_HMI)/3(ACC_State)  "<ACCSve_d_ACC_State_convert>"
  Bus Selector1/8 -> Human_Machine_Interface(ACC_HMI)/9(ACC_DecReq)  "<ACCSve_g_ACC_DecReq_convert>"
  Bus Selector2/1 -> CIPV_Data/1(IMAPva_d_obj_id)  "<IMAPva_d_obj_id_convert>"
  Bus Selector2/2 -> CIPV_Data/2(IMAPva_g_obj_pos_x)  "<IMAPva_g_obj_pos_x_convert>"
  Bus Selector1/6 -> Human_Machine_Interface(ACC_HMI)/7(VelocitySet)  "<ACCSve_d_VelocitySet_convert>"
  In3/1 -> Bus Selector2/1

== system OMAP_ver_MIL10/OMAP_Module/ICA_Direct_G59/ICA_Define ==
  In1 : Inport
  In3 : Inport  Port=2
  In2 : Inport  Port=3
  In4 : Inport  Port=4
  Bus Creator : BusCreator  Inputs=7
  Bus Creator1 : BusCreator  Inputs=6
  Bus Selector : BusSelector  OutputSignals=IMAPve_d_EPS_LKA_State_convert,IMAPve_d_ESC_Veh_Standstill_convert,IMAPve_g_L0_C0_convert,IMAPve_g_L0_C1_convert,IMAPve_g_L0_C2_convert,IMAPve_g_L0_C3_convert,IMAPve_g_R0_C0_convert,IMAPve_g_R0_C1_convert,IMAPve_g_R0_C2_convert,IMAPve_g_R0_C3_convert
  Bus Selector11 : BusSelector  OutputSignals=ICABve_d_ICAMode_convert,ICABve_g_SteerAngleCmd_convert,ICABve_d_LKATorqueReq_convert,ICABve_g_LKATorqueReq_Value_convert,ICABva_d_ICAB2HMI_convert
  Bus Selector2 : BusSelector  OutputSignals=ACCSve_d_ACC_State_convert,ACC_Pop_Up_Message_TJA
  Demux : Demux  Outputs=20
  ICA_EPS : Subsystem
  Subsystem1 : Subsystem
  TH_HMIClb : Subsystem  Description=|
      | Block Name:TH_VFClb
      | No.: THC.05
      | Rev: 00.00.01
      | Update Date: 19-3-28
  Terminator{,1..6} (7 alike) : Terminator
  Out1 : Outport
  Out2 : Outport  Port=2
  wires:
  In2/1 -> Bus Selector/1
  Bus Selector/1 -> ICA_EPS/2(EPSPCEM_stEPSCtlState)  "<IMAPve_d_EPS_LKA_State_convert>"
  TH_HMIClb/1(Out) -> Subsystem1/26(HMI_Clb)  "TH_HMIClb"
  Subsystem1/6(Hands_off_warning) -> Bus Creator1/6  "OMAPve_y_Hands_off_warning_2"
  Subsystem1/5(ISA_Value) -> Bus Creator1/5  "OMAPve_y_ISA_Value_2"
  Subsystem1/4(Vehiclr_Line_Display) -> Bus Creator1/4  "OMAPve_y_Vehicle_Lane_Display_2"
  Subsystem1/1(Dspl_stTxtDspl) -> Bus Creator1/1  "OMAPve_y_ICA_HMI_Txt_Disp_2"
  Subsystem1/3(TSR_Version_Only_Sign_Type) -> Bus Creator1/3  "OMAPve_y_TSR_Vision_Only_Sign_Type_2"
  Subsystem1/2(Dspl_stIconDspl) -> Bus Creator1/2  "OMAPve_y_TJA_status_icon_2"
  Bus Creator1/1 -> Out2/1
  In3/1 -> Terminator/1
  In4/1 -> Bus Selector2/1
  Demux/1 -> Subsystem1/1(EPSRx_stHandOff)  "[1]stHandOff"
  Demux/2 -> Subsystem1/2(EPSRx_stTkOvStChk)  "[2]stTkOvStChk"
  Demux/3 -> Subsystem1/3(L0QI_Opt)  "[3]facmL0QIDisp"
  Demux/4 -> Subsystem1/4(R0QI_Opt)  "[4]facmR0QIDisp"
  Demux/5 -> Subsystem1/6(L0Type_Opt)  "[5]L0Type_Opt"
  Demux/6 -> Subsystem1/7(R0Type_Opt)  "[6]R0Type_Opt"
  Demux/7 -> Subsystem1/8(stTHState)  "[7]stTHState"
  Demux/8 -> Subsystem1/11(stTHFKeyStt)  "[8]stTHFKeyStt"
  Demux/9 -> Subsystem1/13(stTHAutRydEnaFlg)  "[9]THAutRydEnaFlg"
  Demux/10 -> Subsystem1/14(stSWALimFlg)  "[10]stSWALimFlg"
  Demux/11 -> Subsystem1/15(stTHMode)  "[11]stTHMode"
  Demux/12 -> Subsystem1/17(stLCScene)  "[12]stLCScene"
  Demux/15 -> Subsystem1/12(HMI_tfAddVocCmd)  "[15]tfAddVocCmd"
  Demux/16 -> Subsystem1/16(stLCRMode)
  Bus Selector2/2 -> Subsystem1/10(ACC_HMI_Txt_Disp)  "<ACC_Pop_Up_Message_TJA>"
  Bus Selector2/1 -> Subsystem1/9(ACC_State)  "<ACCSve_d_ACC_State_convert>"
  Bus Selector/2 -> Subsystem1/5(VehMovRx_VehicleStationary)  "<IMAPve_d_ESC_Veh_Standstill_convert>"
  Bus Selector/3 -> Subsystem1/18(L0C0_Org)  "<IMAPve_g_L0_C0_convert>"
  Bus Selector/4 -> Subsystem1/19(L0C1_Org)  "<IMAPve_g_L0_C1_convert>"
  Bus Selector/5 -> Subsystem1/20(L0C2_Org)  "<IMAPve_g_L0_C2_convert>"
  Bus Selector/6 -> Subsystem1/21(L0C3_Org)  "<IMAPve_g_L0_C3_convert>"
  Bus Selector/7 -> Subsystem1/22(R0C0_Org)  "<IMAPve_g_R0_C0_convert>"
  Bus Selector/8 -> Subsystem1/23(R0C1_Org)  "<IMAPve_g_R0_C1_convert>"
  Bus Selector/9 -> Subsystem1/24(R0C2_Org)  "<IMAPve_g_R0_C2_convert>"
  Bus Selector/10 -> Subsystem1/25(R0C3_Org)  "<IMAPve_g_R0_C3_convert>"
  In1/1 -> Bus Selector11/1
  Bus Selector11/2 -> Bus Creator/5  "<ICABve_g_SteerAngleCmd_convert>"
  Bus Selector11/4 -> Bus Creator/7  "<ICABve_g_LKATorqueReq_Value_convert>"
  Bus Selector11/5 -> Demux/1  "<ICABva_d_ICAB2HMI_convert>"
  Bus Selector11/1 -> ICA_EPS/1(EPSPCEM_stICAMode)  "<ICABve_d_ICAMode_convert>"
  Bus Selector11/3 -> Bus Creator/6  "<ICABve_d_LKATorqueReq_convert>"
  ICA_EPS/1(stEPS_State_Ctl_CMD) -> Bus Creator/1  "OMAPve_y_General_state_of_LKA_function3F2_2"
  ICA_EPS/3(LKA_OR_LPA_REQ) -> Bus Creator/3  "OMAPve_y_Permit_to_know_if_LKA_or_LPA3F2_2"
  ICA_EPS/4(ICA_MODE) -> Bus Creator/4
  ICA_EPS/2(LKA_TRQ_FACT_REQ) -> Bus Creator/2  "OMAPve_g_Coefficient_toregulate_EPS_2"
  Bus Creator/1 -> Out1/1
  Demux/13 -> Terminator1/1  "[13]stLCMode"
  Demux/14 -> Terminator2/1  "[14]stLFState"
  Demux/17 -> Terminator3/1
  Demux/18 -> Terminator4/1
  Demux/19 -> Terminator5/1
  Demux/20 -> Terminator6/1

== system OMAP_ver_MIL10/OMAP_Module/ACCS_Direct/ACCS_Define/ACC_State_Synthesis(ACC_SS) ==
  Input_ACCS : Inport
  Bus Selector : BusSelector  OutputSignals=Deceleration_setpoint_device,TminDownGear,TminUpGear,StAcvTqWhlPTPotReq,PotACCTqReq,Function_Acc_status,ACCTqReq,Powertrain_torquewheel_request,TYPE_RAPPORT,MDD_Decelerationcontrol_request,MDD_deceleration_type,Power_steering_power_cut3F2
  Bus Selector2 : BusSelector  OutputSignals=ACCSve_d_ACC_State_convert
  Compare To Constant1 : simulink/Logic and Bit Operations/Compare To Constant  relop===  const=0  OutDataTypeStr=boolean
  Compare To Constant2 : simulink/Logic and Bit Operations/Compare To Constant  relop===  const=1  OutDataTypeStr=boolean
  Compare To Constant5 : simulink/Logic and Bit Operations/Compare To Constant  relop===  const=2  OutDataTypeStr=boolean
  Compare To Constant6 : simulink/Logic and Bit Operations/Compare To Constant  relop===  const=3  OutDataTypeStr=boolean
  Compare To Constant7 : simulink/Logic and Bit Operations/Compare To Constant  relop===  const=15  OutDataTypeStr=boolean
  If Action Subsystem2 : Subsystem  TreatAsAtomicUnit=on
  If Action Subsystem3 : Subsystem  TreatAsAtomicUnit=on
  If1 : If  IfExpression=u1 == 1
  Logical Operator1 : Logic  Operator=OR  Inputs=5  AllPortsSameDT=off  OutDataTypeStr=boolean
  Merge : Merge
  ACC_Control_Signal : Outport
  tag scope: ob_ACC_ACCTqReq=global, ob_ACC_Deceleration_setpoint_device=global, ob_ACC_Function_Acc_status=global, ob_ACC_MDD_Decelerationcontrol_request=global, ob_ACC_MDD_deceleration_type=global, ob_ACC_PotACCTqReq=global, ob_ACC_Power_steering_power_cut3F2=global, ob_ACC_Powertrain_torquewheel_request=global, ob_ACC_StAcvTqWhlPTPotReq=global, ob_ACC_TYPE_RAPPORT=global, ob_ACC_TminDownGear=global, ob_ACC_TminUpGear=global
  wires:
  Input_ACCS/1 -> Bus Selector2/1, If Action Subsystem3/1(ACT_Control_Signal)
  Bus Selector/12 -> [ob_ACC_Power_steering_power_cut3F2]  "<Power_steering_power_cut3F2>"
  Bus Selector/11 -> [ob_ACC_MDD_deceleration_type]  "<MDD_deceleration_type>"
  Bus Selector/10 -> [ob_ACC_MDD_Decelerationcontrol_request]  "<MDD_Decelerationcontrol_request>"
  Bus Selector/9 -> [ob_ACC_TYPE_RAPPORT]  "<TYPE_RAPPORT>"
  Bus Selector/8 -> [ob_ACC_Powertrain_torquewheel_request]  "<Powertrain_torquewheel_request>"
  Bus Selector/7 -> [ob_ACC_ACCTqReq]  "<ACCTqReq>"
  Bus Selector/6 -> [ob_ACC_Function_Acc_status]  "<Function_Acc_status>"
  Bus Selector/5 -> [ob_ACC_PotACCTqReq]  "<PotACCTqReq>"
  Bus Selector/4 -> [ob_ACC_StAcvTqWhlPTPotReq]  "<StAcvTqWhlPTPotReq>"
  Bus Selector/3 -> [ob_ACC_TminUpGear]  "<TminUpGear>"
  Bus Selector/2 -> [ob_ACC_TminDownGear]  "<TminDownGear>"
  Bus Selector/1 -> [ob_ACC_Deceleration_setpoint_device]  "<Deceleration_setpoint_device>"
  Merge/1 -> ACC_Control_Signal/1, Bus Selector/1  "Control_Ouput"
  If Action Subsystem3/1(Control_Ouput) -> Merge/2
  If Action Subsystem2/1(Control_Ouput) -> Merge/1
  If1/2 -> If Action Subsystem3/Action
  If1/1 -> If Action Subsystem2/Action
  Logical Operator1/1 -> If1/1
  Compare To Constant7/1 -> Logical Operator1/5
  Compare To Constant6/1 -> Logical Operator1/4
  Compare To Constant5/1 -> Logical Operator1/3
  Compare To Constant1/1 -> Logical Operator1/1
  Compare To Constant2/1 -> Logical Operator1/2
  Bus Selector2/1 -> Compare To Constant1/1, Compare To Constant2/1, Compare To Constant5/1, Compare To Constant6/1, Compare To Constant7/1, If Action Subsystem2/1(In1)  "<ACCSve_d_ACC_State_convert>"

== system OMAP_ver_MIL10/OMAP_Module/ACCS_Direct/ACCS_Define/Human_Machine_Interface(ACC_HMI) ==
  CIPV_ID_Longitudinal_Distance : Inport
  CIPV_ID : Inport  Port=2
  ACC_State : Inport  Port=3
  ACCActive_Signal : Inport  Port=4
  ACC_ICA_Flag : Inport  Port=5
  HeadWaySet : Inport  Port=6
  VelocitySet : Inport  Port=7
  ACC_go_request : Inport  Port=8
  ACC_DecReq : Inport  Port=9
  Bus Selector : BusSelector  OutputSignals=ACC_Vehicle_Icon_Display,ACC_Set_Speed_Display,ACC_DesiredHeadway_Icon_Basic,RVVACC_Vehiclespeed_request_type
  Gain : Gain  OutDataTypeStr=uint8
  Gain1 : Gain  OutDataTypeStr=uint8
  Subsystem : Subsystem
  Subsystem9 : Subsystem
  Text_PopUp : Subsystem
  ACC_DesiredHeadway_Display : Outport
  ACC_DesiredHeadway_Icon_Basic : Outport  Port=2
  ACC_Desired_Set_Speed : Outport  Port=3
  ACC_Set_Speed_Display : Outport  Port=4
  ACC_Vehicle_Icon_Display : Outport  Port=5
  RVVACC_Vehiclespeed_request_type : Outport  Port=6
  ACC_Pop_Up_Message : Outport  Port=7
  ACC_HMI_TgDisp_Flag : Outport  Port=8
  TARGET_POSITION : Outport  Port=9
  ACC_Pop_Up_Message_TJA : Outport  Port=10
  wires:
  VelocitySet/1 -> Gain/1, Subsystem9/3(VelocitySet)
  HeadWaySet/1 -> Gain1/1
  Subsystem9/1(Out1) -> Bus Selector/1
  Gain/1 -> ACC_Desired_Set_Speed/1  "ACC_Desired_Set_Speed"
  CIPV_ID_Longitudinal_Distance/1 -> Subsystem/1(Distance)
  Subsystem/2(TgDisp_Flag) -> ACC_HMI_TgDisp_Flag/1  "ACC_HMI_TgDisp_Flag"
  Subsystem/1(TARGET_POSITION) -> TARGET_POSITION/1  "TARGET_POSITION"
  CIPV_ID/1 -> Subsystem/2(CIPV_ID)
  Gain1/1 -> ACC_DesiredHeadway_Display/1  "ACC_DesiredHeadway_Display"
  Text_PopUp/1(For4F7) -> ACC_Pop_Up_Message/1  "ACC_Pop_Up_Message"
  Bus Selector/1 -> ACC_Vehicle_Icon_Display/1  "<ACC_Vehicle_Icon_Display>"
  Bus Selector/3 -> ACC_DesiredHeadway_Icon_Basic/1  "<ACC_DesiredHeadway_Icon_Basic>"
  Bus Selector/4 -> RVVACC_Vehiclespeed_request_type/1  "<RVVACC_Vehiclespeed_request_type>"
  Bus Selector/2 -> ACC_Set_Speed_Display/1  "<ACC_Set_Speed_Display>"
  ACCActive_Signal/1 -> Text_PopUp/3(ACCActive_Signal)
  Text_PopUp/2(ForTJA) -> ACC_Pop_Up_Message_TJA/1  "ACC_Pop_Up_Message_TJA"
  ACC_go_request/1 -> Text_PopUp/4(go_request)
  ACC_State/1 -> Subsystem9/1(ACC_State), Text_PopUp/1(ACC_State), Subsystem/3(ACC_State)
  ACC_ICA_Flag/1 -> Subsystem9/2(ACCICA_Flag), Text_PopUp/2(ACCICA_Flag)
  ACC_DecReq/1 -> Text_PopUp/5(ACC_DecReq)

== system OMAP_ver_MIL10/OMAP_Module/ICA_Direct_G59/ICA_Define/ICA_EPS ==
  EPSPCEM_stICAMode : Inport
  EPSPCEM_stEPSCtlState : Inport  Port=2
  Data Type Conversion : DataTypeConversion  OutDataTypeStr=uint16
  Data Type Conversion1 : DataTypeConversion  OutDataTypeStr=single
  Data Type Conversion2 : DataTypeConversion  OutDataTypeStr=uint16
  EPS_Ctr_Disable : Subsystem  TreatAsAtomicUnit=on
  EPS_Ctr_Enable : Subsystem  TreatAsAtomicUnit=on
  If1 : If  IfExpression=u1~= 0
  Merge1 : Merge
  Merge2 : Merge
  Merge3 : Merge
  stEPS_State_Ctl_CMD : Outport
  LKA_TRQ_FACT_REQ : Outport  Port=2
  LKA_OR_LPA_REQ : Outport  Port=3
  ICA_MODE : Outport  Port=4
  wires:
  Merge1/1 -> Data Type Conversion/1
  EPSPCEM_stEPSCtlState/1 -> EPS_Ctr_Enable/1(stEPSCtlState), EPS_Ctr_Disable/1(stEPSCtlState)
  EPS_Ctr_Enable/1(stEPSCtlCMD) -> Merge1/1
  If1/2 -> EPS_Ctr_Disable/Action
  EPS_Ctr_Enable/2(LKA_TRQ_FACT_REQ) -> Merge2/1
  EPS_Ctr_Disable/2(LKA_TRQ_FACT_REQ) -> Merge2/2
  Merge2/1 -> Data Type Conversion1/1
  EPSPCEM_stICAMode/1 -> ICA_MODE/1, If1/1
  Data Type Conversion1/1 -> LKA_TRQ_FACT_REQ/1  "LKA_TRQ_FACT_REQ"
  EPS_Ctr_Disable/1(stEPSCtlCMD) -> Merge1/2
  If1/1 -> EPS_Ctr_Enable/Action
  Data Type Conversion/1 -> stEPS_State_Ctl_CMD/1
  EPS_Ctr_Enable/3(LKA_OR_LPA_REQ) -> Merge3/1
  Data Type Conversion2/1 -> LKA_OR_LPA_REQ/1
  Merge3/1 -> Data Type Conversion2/1
  EPS_Ctr_Disable/3(LKA_OR_LPA_REQ) -> Merge3/2

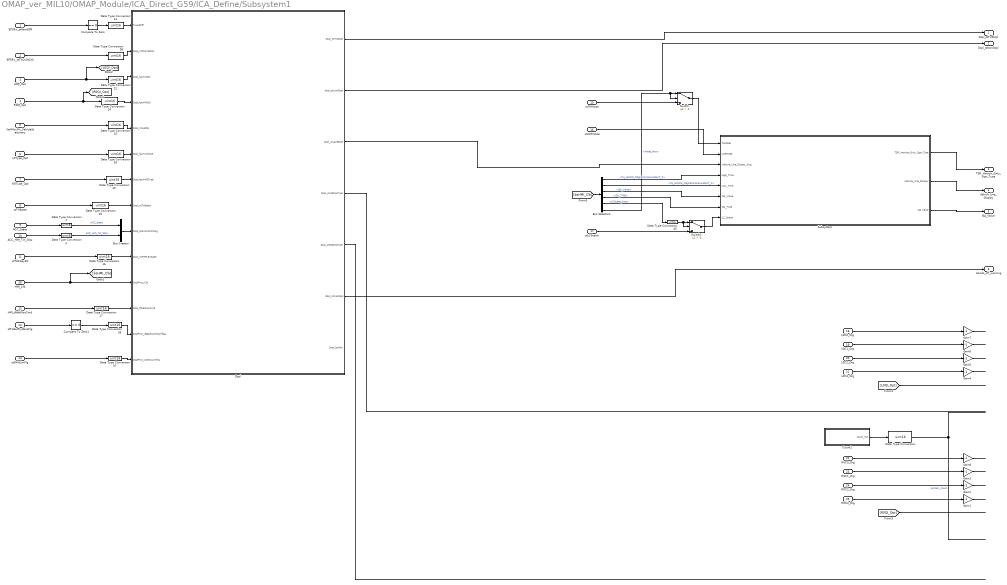
== system OMAP_ver_MIL10/OMAP_Module/ICA_Direct_G59/ICA_Define/Subsystem1 ==
  EPSRx_stHandOff : Inport
  EPSRx_stTkOvStChk : Inport  Port=2
  L0QI_Opt : Inport  Port=3
  R0QI_Opt : Inport  Port=4
  VehMovRx_VehicleStationary : Inport  Port=5
  L0Type_Opt : Inport  Port=6
  R0Type_Opt : Inport  Port=7
  stTHState : Inport  Port=8
  ACC_State : Inport  Port=9
  ACC_HMI_Txt_Disp : Inport  Port=10
  stTHFKeyStt : Inport  Port=11
  HMI_tfAddVocCmd : Inport  Port=12
  stTHAutRydEnaFlg : Inport  Port=13
  stSWALimFlg : Inport  Port=14
  stTHMode : Inport  Port=15
  stLCRMode : Inport  Port=16
  stLCScene : Inport  Port=17
  L0C0_Org : Inport  Port=18
  L0C1_Org : Inport  Port=19
  L0C2_Org : Inport  Port=20
  L0C3_Org : Inport  Port=21
  R0C0_Org : Inport  Port=22
  R0C1_Org : Inport  Port=23
  R0C2_Org : Inport  Port=24
  R0C3_Org : Inport  Port=25
  HMI_Clb : Inport  Port=26
  Bus Creator : BusCreator  Inputs=2
  Bus Selector1 : BusSelector  OutputSignals=TH_HMIClb_tiDgrdIconWarnHiDurT_C,TH_HMIClb_tiDgrdIconWarnLoDurT_C,ISA_Value,ISA_TYPE,LCScene_tmp,Mode_tmp
  Compare To Zero : simulink/Logic and Bit Operations/Compare To Zero  relop===  OutDataTypeStr=boolean
  Compare To Zero1 : simulink/Logic and Bit Operations/Compare To Zero  relop===  OutDataTypeStr=boolean
  Count1 : MATLAB Function  TreatAsAtomicUnit=on
  Data Type Conversion{,14..17,22,24,35..40,45} (14 alike) : DataTypeConversion  OutDataTypeStr=uint16
  Data Type Conversion1 : DataTypeConversion  OutDataTypeStr=uint8
  Data Type Conversion2 : DataTypeConversion  OutDataTypeStr=uint8
  Dspl : Subsystem
  Gain{1..8} (8 alike) : Gain  Gain=-1  OutDataTypeStr=single
  Subsystem : Subsystem
  Switch : Switch  Criteria=u2 > Threshold
  Switch1 : Switch  Criteria=u2 > Threshold
  Dspl_stTxtDspl : Outport
  Dspl_stIconDspl : Outport  Port=2
  TSR_Version_Only_Sign_Type : Outport  Port=3
  Vehiclr_Line_Display : Outport  Port=4
  ISA_Value : Outport  Port=5
  Hands_off_warning : Outport  Port=6
  wires:
  stLCRMode/1 -> Subsystem/2(LCRMode)
  R0C3_Org/1 -> Gain1/1
  L0C0_Org/1 -> Gain7/1
  stTHFKeyStt/1 -> Data Type Conversion16/1
  [L0QI_Opt] -> ?
  Dspl/6(Dspl_stVocDspl) -> Hands_off_warning/1
  stLCScene/1 -> Switch1/3
  stTHMode/1 -> Switch/3
  L0QI_Opt/1 -> [L0QI_Opt], Data Type Conversion22/1
  stTHAutRydEnaFlg/1 -> Compare To Zero1/1
  stTHState/1 -> Data Type Conversion35/1
  stSWALimFlg/1 -> Data Type Conversion37/1
  [R0QI_Opt] -> ?
  R0C0_Org/1 -> Gain8/1
  L0C2_Org/1 -> Gain5/1
  R0Type_Opt/1 -> Data Type Conversion40/1
  VehMovRx_VehicleStationary/1 -> Data Type Conversion15/1
  Data Type Conversion24/1 -> Dspl/4(Dspl_facmR0Ql)
  R0QI_Opt/1 -> [R0QI_Opt], Data Type Conversion24/1
  R0C1_Org/1 -> Gain3/1
  Compare To Zero1/1 -> Data Type Conversion36/1
  Data Type Conversion39/1 -> Dspl/6(Dspl_facmL0Type)
  Data Type Conversion37/1 -> Dspl/14(DsplPrcs_stSWALimFlg)
  L0C3_Org/1 -> Gain4/1
  Data Type Conversion17/1 -> Dspl/12(Dspl_tfAddVocCmd)
  Bus Selector1/5 -> Data Type Conversion45/1  "<LCScene_tmp>"
  Data Type Conversion16/1 -> Dspl/10(Dspl_stTHFKeyState)
  EPSRx_stTkOvStChk/1 -> Data Type Conversion38/1
  [bsHMI_Clb] -> Bus Selector1/1
  Data Type Conversion45/1 -> Switch1/2, Switch1/1
  Data Type Conversion36/1 -> Dspl/13(DsplPrcs_dDgrdIconWarnflag)
  HMI_Clb/1 -> [bsHMI_Clb], Dspl/11(DsplPrcs_CIb)
  Data Type Conversion40/1 -> Dspl/7(Dspl_facmR0Type)
  Bus Selector1/2 -> Subsystem/5(Low_Time)  "<TH_HMIClb_tiDgrdIconWarnLoDurT_C>"
  Count1/1(count_out) -> Data Type Conversion/1
  Compare To Zero/1 -> Data Type Conversion14/1
  Dspl/3(Dspl_stLaneDspl) -> Subsystem/3(Vehicle_Line_Display_Org)
  Switch/1 -> Subsystem/1(THMode)
  Data Type Conversion22/1 -> Dspl/3(Dspl_facmL0Ql)
  EPSRx_stHandOff/1 -> Compare To Zero/1
  Data Type Conversion15/1 -> Dspl/5(Dspl_stVehSty)
  Dspl/5(Dspl_stR0DispType) -> ?
  Data Type Conversion35/1 -> Dspl/8(Dspl_stTHState)
  Data Type Conversion14/1 -> Dspl/1(TxHndOff)
  Dspl/4(Dspl_stL0DispType) -> ?
  L0C1_Org/1 -> Gain6/1
  L0Type_Opt/1 -> Data Type Conversion39/1
  Bus Selector1/1 -> Subsystem/4(High_Time)  "<TH_HMIClb_tiDgrdIconWarnHiDurT_C>"
  Gain2/1 -> ?
  Gain3/1 -> ?
  Gain7/1 -> ?
  R0C2_Org/1 -> Gain2/1
  Gain6/1 -> ?
  Gain5/1 -> ?
  Gain8/1 -> ?
  Switch1/1 -> Subsystem/8(LC_Scene)
  Gain1/1 -> ?
  HMI_tfAddVocCmd/1 -> Data Type Conversion17/1
  Subsystem/1(TSR_Version_Only_Sign_Type) -> TSR_Version_Only_Sign_Type/1
  Bus Selector1/3 -> Subsystem/6(ISA_Value)  "<ISA_Value>"
  Subsystem/3(ISA Value) -> ISA_Value/1
  Bus Selector1/4 -> Subsystem/7(ISA_Type)  "<ISA_TYPE>"
  Subsystem/2(Vehicle_Line_Display) -> Vehiclr_Line_Display/1
  Data Type Conversion38/1 -> Dspl/2(Dspl_stTkOvStChk)
  Data Type Conversion/1 -> ?  "System_Count"
  Gain4/1 -> ?
  Bus Selector1/6 -> Switch/2, Switch/1  "<Mode_tmp>"
  Bus Creator/1 -> Dspl/9(Dspl_bsFromFMCMsg)
  Data Type Conversion2/1 -> Bus Creator/2  "ACC_HMI_Txt_Disp"
  Data Type Conversion1/1 -> Bus Creator/1  "ACC_State"
  ACC_HMI_Txt_Disp/1 -> Data Type Conversion2/1
  ACC_State/1 -> Data Type Conversion1/1
  Dspl/1(Dspl_stTxtDspl) -> Dspl_stTxtDspl/1
  Dspl/2(Dspl_stIconDspl) -> Dspl_stIconDspl/1
